simulink model "third"  (R2020a)
settings: Solver=VariableStepAuto  StartTime=0.0  StopTime=10.0  RelTol=1e-3
model workspace (MAT data in the model file):
  Kd = Simulink.Parameter
  Kd.Value = 50
  Kd.DataType = 'auto'
  Kd.Dimensions = [1 1]
  Ki = Simulink.Parameter
  Ki.Value = 300
  Ki.DataType = 'auto'
  Ki.Dimensions = [1 1]
  Kp = Simulink.Parameter
  Kp.Value = 350
  Kp.DataType = 'auto'
  Kp.Dimensions = [1 1]
  b = Simulink.Parameter
  b.Value = 50
  b.DataType = 'auto'
  b.Dimensions = [1 1]
  m = Simulink.Parameter
  m.Value = 1000
  m.DataType = 'auto'
  m.Dimensions = [1 1]
settings Model: Creator=Admin  LastModifiedBy=Admin

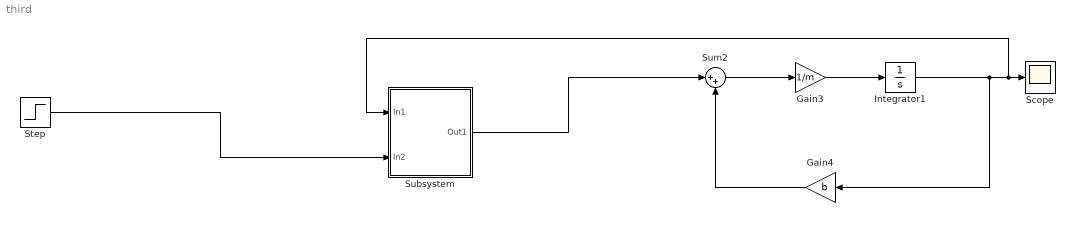
== system third ==
  Gain3 : Gain  Gain=1/m
  Gain4 : Gain  Gain=b
  Integrator1 : Integrator
  Scope : Scope
  Step : Step  SampleTime=0
  Subsystem : Subsystem  TreatAsAtomicUnit=on
  Sum2 : Sum  Inputs=|++
  wires:
  Sum2/1 -> Gain3/1
  Gain3/1 -> Integrator1/1
  Integrator1/1 -> Subsystem/1(In1), Scope/1, Gain4/1
  Gain4/1 -> Sum2/2
  Step/1 -> Subsystem/2(In2)
  Subsystem/1(Out1) -> Sum2/1

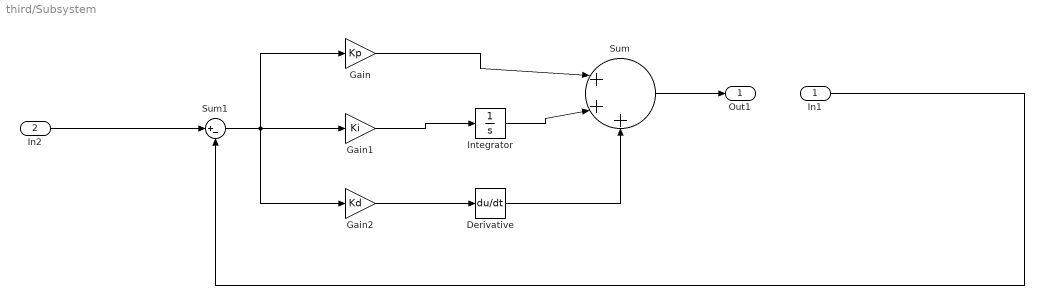
== system third/Subsystem ==
  In1 : Inport
  In2 : Inport  Port=2
  Derivative : Derivative
  Gain : Gain  Gain=Kp
  Gain1 : Gain  Gain=Ki
  Gain2 : Gain  Gain=Kd
  Integrator : Integrator
  Sum : Sum  Inputs=|+++
  Sum1 : Sum  Inputs=|+-
  Out1 : Outport
  wires:
  Gain1/1 -> Integrator/1
  Sum1/1 -> Gain2/1, Gain/1, Gain1/1
  In1/1 -> Sum1/2
  Derivative/1 -> Sum/3
  Gain2/1 -> Derivative/1
  Sum/1 -> Out1/1
  Integrator/1 -> Sum/2
  Gain/1 -> Sum/1
  In2/1 -> Sum1/1
